simulink model "youbot_no_encoders_joystick_control"  (R2013b)
settings: Solver=ode3  StartTime=0.0  StopTime=inf  FixedStep=0.01  RelTol=1e-3
libraries: vrlib x1, robotica x1
settings Model: Creator=student  LastModifiedBy=student

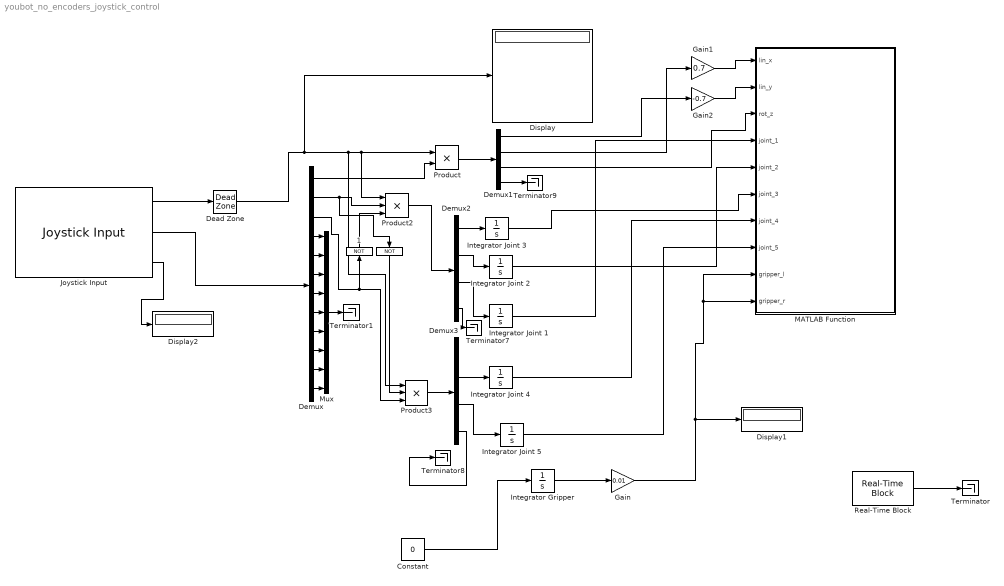
== system youbot_no_encoders_joystick_control ==
  " " : Logic  Operator=NOT  AllPortsSameDT=off  OutDataTypeStr=boolean
  " 1" : Logic  Operator=NOT  AllPortsSameDT=off  OutDataTypeStr=boolean
  Constant : Constant  Value=0
  Dead Zone : DeadZone  LowerValue=-0.1  UpperValue=0.1  SaturateOnIntegerOverflow=on
  Demux : Demux  Outputs=12
  Demux1 : Demux
  Demux2 : Demux
  Demux3 : Demux
  Display : Display
  Display1 : Display
  Display2 : Display
  Gain : Gain  Gain=0.01
  Gain1 : Gain  Gain=0.7
  Gain2 : Gain  Gain=-0.7
  Integrator Gripper : Integrator  LimitOutput=on  UpperSaturationLimit=1  LowerSaturationLimit=0
  "Integrator Joint 5 " : Integrator  InitialCondition=0.12  LimitOutput=on  UpperSaturationLimit=5.64  LowerSaturationLimit=0.12
  "Integrator Joint 1 " : Integrator  InitialCondition=0.02  LimitOutput=on  UpperSaturationLimit=5.84  LowerSaturationLimit=0.02
  Integrator Joint 2 : Integrator  InitialCondition=0.02  LimitOutput=on  UpperSaturationLimit=2.61  LowerSaturationLimit=0.02
  "Integrator Joint 3 " : Integrator  InitialCondition=-0.02  LimitOutput=on  UpperSaturationLimit=-0.02  LowerSaturationLimit=-5.02
  Integrator Joint 4 : Integrator  InitialCondition=0.03  LimitOutput=on  UpperSaturationLimit=3.42  LowerSaturationLimit=0.03
  Joystick Input : vrlib/Joystick Input  joyid=1  adjustports=on  forcefeed=off
  MATLAB Function : MATLAB Function  StartFcn=|  StopFcn=|  TreatAsAtomicUnit=on  mask{youbot_IP=192.168.65.59, youbot_port=11311}
      StartFcn=|
      | %ros_node = rosmatlab.node('KUKA_SIMULINK_CONTROL','192.168.65.59',11311);          
      |  ros_node = rosmatlab.node('KUKA_SIMULINK_CONTROL',youbot_ip, youbot_port);          
      | 
      | % Base                                        
      | 
      |     publisher_na_kuko = rosmatlab.publisher('/cmd_vel','geometry_msgs/Twist',ros_node);                                     
      |     kuka_message = rosmatlab.message('geometry_msgs/Twist',ros_node);                                                       
      |     kuka_message.getLinear.setX(0.0);                                                                                       
      |     kuka_message.getLinear.setY(0);                                                                                         
      |     kuka_message.getLinear.setZ(0);                                                                                         
      |     kuka_message.getAngular.setX(0);                                                                                        
      |     kuka_message.getAngular.setY(0);                                                                                        
      |     kuka_message.getAngular.setZ(0);                                                                                        
      |     publisher_na_kuko.publish(kuka_message);                                                                                
      | 
      | % Arm
      |                                                                                                                             
      | publisher_kuka_arm = rosmatlab.publisher('/arm_1/arm_controller/position_command','brics_actuator/JointPositions',ros_node);
      |                                                                                                                             
      | arm_kuka_message = rosmatlab.message('brics_actuator/JointPositions', ros_node);                                            
      |                                                                                                                             
      | arm_header_message = rosmatlab.message('brics_actuator/Poison', ros_node);                                                  
      |                                                                                                                             
      | joint_1_message =  rosmatlab.message('brics_actuator/JointValue', ros_node);                                                
      |                                                                                                                             
      | joint_2_message= rosmatlab.message('brics_actuator/JointValue', ros_node);                                                  
      |                                                                                                                             
      | joint_3_message = rosmatlab.message('brics_actuator/JointValue', ros_node);                                                 
      |                                                                                                                             
      | joint_4_message = rosmatlab.message('brics_actuator/JointValue', ros_node);                                                 
      |                                                                                                                             
      | joint_5_message = rosmatlab.message('brics_actuator/JointValue', ros_node);                                                 
      |                                                                                                                             
      | arm_header_message.setDescription('Pozdrav iz Simulinka');                                                                  
      | arm_header_message.setOriginator('Simulink');                                                                               
      | arm_header_message.setQos(0.0);                                                                                             
      | arm_kuka_message.setPoisonStamp(arm_header_message);                                                                        
      |                                                                                                                             
      | joint_1_message.setJointUri('arm_joint_1');                                                                                 
      | joint_1_message.setUnit('rad');                                                                                             
      | joint_1_message.setValue(0.02);                                                                                                
      |                                                                                                                             
      | joint_2_message.setJointUri('arm_joint_2');                                                                                 
      | joint_2_message.setUnit('rad');                                                                                             
      | joint_2_message.setValue(0.02);                                                                                                
      |                                                                                                                             
      | joint_3_message.setJointUri('arm_joint_3');                                                                                 
      | joint_3_message.setUnit('rad');                                                                                             
      | joint_3_message.setValue(-0.02);                                                                                                
      |                                                                                                                             
      | joint_4_message.setJointUri('arm_joint_4');                                                                                 
      | joint_4_message.setUnit('rad');                                                                                             
      | joint_4_message.setValue(0.023);                                                                                                
      |                                                                                                                             
      | joint_5_message.setJointUri('arm_joint_5');                                                                                 
      | joint_5_message.setUnit('rad');                                                                                             
      | joint_5_message.setValue(0.12);                                                                                                
      |                                                                                                                             
      | arm_kuka_message.getPositions.add(joint_1_message);                                                                         
      | arm_kuka_message.getPositions.add(joint_2_message);                                                                         
      | arm_kuka_message.getPositions.add(joint_3_message);                                                                         
      | arm_kuka_message.getPositions.add(joint_4_message);                                                                         
      | arm_kuka_message.getPositions.add(joint_5_message);                                                                         
      |                                                                                                                             
      | publisher_kuka_arm.publish(arm_kuka_message);     
      | 
      | % Gripper
      | 
      | gripper_publisher = rosmatlab.publisher('/arm_1/gripper_controller/position_command','brics_actuator/JointPositions',ros_node);
      | 
      | gripper_message = rosmatlab.message('brics_actuator/JointPositions', ros_node);
      | gripper_header_message = rosmatlab.message('brics_actuator/Poison', ros_node);
      | gripper_L_message =  rosmatlab.message('brics_actuator/JointValue', ros_node);
      | gripper_R_message= rosmatlab.message('brics_actuator/JointValue', ros_node);
      | 
      | gripper_header_message.setDescription('Hello Simulink.  Gripper greets you');
      | gripper_header_message.setOriginator('Simulink');
      | gripper_header_message.setQos(0.0);
      | gripper_message.setPoisonStamp(gripper_header_message);
      | 
      | gripper_L_message.setJointUri('gripper_finger_joint_l');
      | gripper_L_message.setUnit('m');
      | gripper_L_message.setValue(0);
      | 
      | gripper_R_message.setJointUri('gripper_finger_joint_r');
      | gripper_R_message.setUnit('m');
      | gripper_R_message.setValue(0);
      | 
      | gripper_message.getPositions.add(gripper_L_message);
      | gripper_message.getPositions.add(gripper_R_message);
      | 
      | gripper_publisher.publish(gripper_message);
      StopFcn=|
      | kuka_message.getLinear.setX(0);         
      | kuka_message.getLinear.setY(0);         
      | kuka_message.getLinear.setZ(0);         
      | kuka_message.getAngular.setX(0);        
      | kuka_message.getAngular.setY(0);        
      | kuka_message.getAngular.setZ(0);        
      | publisher_na_kuko.publish(kuka_message);
      | ros_node.delete                         
      | 
      | clear arm_header_message;
      | clear arm_kuka_message;
      | clear gripper_L_message;
      | clear gripper_R_message;
      | clear gripper_header_message;
      | clear gripper_message;
      | clear gripper_publisher;
      | clear joint_1_message;
      | clear joint_2_message;
      | clear joint_3_message;
      | clear joint_4_message;
      | clear joint_5_message;
      | 
      | clear kuka_message;
      | clear publisher_na_kuko;
      | clear publisher_kuka_arm;
      | 
      | 
      | clear youbot_ip;
      | clear youbot_port;
      | 
      | clear ros_node;
      mask prompts: youbot_IP "Youbot IP address"; youbot_port "Youbot port"
      mask help: Enter the Kuka Youbot IP address and ros core port number.
      mask init:
      | disp('Entered kuka youbot block mask initialization');
      | assignin('base','youbot_ip',youbot_IP);
      | assignin('base','youbot_port',youbot_port);
  Mux : Mux  Inputs=9
  Product : Product
  Product2 : Product  Inputs=3
  Product3 : Product  Inputs=3
  Real-Time Block : robotica/Utilities blocks/Real-Time Block  sync_type=Fixed  sync_time=0.01
  Terminator{,1,7..9} (5 alike) : Terminator
  wires:
  Real-Time Block/1 -> Terminator/1
  Joystick Input/1 -> Dead Zone/1
  Joystick Input/3 -> Display2/1
  Joystick Input/2 -> Demux/1
  Demux/1 -> Product/2
  Demux/2 -> " "/1, Product2/2
  Demux/3 -> Product3/3, " 1"/1
  Demux/4 -> Mux/1
  Demux/5 -> Mux/2
  Demux/6 -> Mux/3
  Demux/7 -> Mux/4
  Demux/8 -> Mux/5
  Demux/9 -> Mux/6
  Demux/10 -> Mux/7
  Demux/11 -> Mux/8
  Demux/12 -> Mux/9
  Mux/1 -> Terminator1/1
  Demux1/3 -> MATLAB Function/3(rot_z)
  Demux1/2 -> Gain1/1
  Demux1/1 -> Gain2/1
  Constant/1 -> Integrator Gripper/1
  Integrator Gripper/1 -> Gain/1
  Gain/1 -> MATLAB Function/9(gripper_l), MATLAB Function/10(gripper_r), Display1/1
  Product/1 -> Demux1/1
  Gain1/1 -> MATLAB Function/1(lin_x)
  Gain2/1 -> MATLAB Function/2(lin_y)
  Dead Zone/1 -> Display/1, Product3/1, Product2/1, Product/1
  Product2/1 -> Demux2/1
  Demux2/3 -> "Integrator Joint 1 "/1
  "Integrator Joint 1 "/1 -> MATLAB Function/4(joint_1)
  Demux2/2 -> Integrator Joint 2/1
  Integrator Joint 2/1 -> MATLAB Function/5(joint_2)
  Demux2/1 -> "Integrator Joint 3 "/1
  "Integrator Joint 3 "/1 -> MATLAB Function/6(joint_3)
  " "/1 -> Product3/2
  " 1"/1 -> Product2/3
  Product3/1 -> Demux3/1
  Demux3/2 -> Integrator Joint 4/1
  Integrator Joint 4/1 -> MATLAB Function/7(joint_4)
  Demux2/4 -> Terminator7/1
  Demux3/3 -> "Integrator Joint 5 "/1
  "Integrator Joint 5 "/1 -> MATLAB Function/8(joint_5)
  Demux3/4 -> Terminator8/1
  Demux1/4 -> Terminator9/1

== matlab function youbot_no_encoders_joystick_control/MATLAB Function ==
  data: lin_x input; lin_y input; rot_z input; joint_1 input; joint_2 input; joint_3 input; joint_4 input; joint_5 input; gripper_l input; gripper_r input
function youbot_control_no_encoders(lin_x,lin_y,rot_z,joint_1,joint_2,joint_3,joint_4,joint_5,gripper_l,gripper_r)

persistent lin_x_old lin_y_old rot_z_old;
persistent joint_1_old joint_2_old joint_3_old joint_4_old joint_5_old ;
persistent gripper_l_old gripper_r_old ; 

if isempty(lin_x_old)  % all initialized at first step
    lin_x_old = 0;
    lin_y_old = 0;
    rot_z_old = 0;
    joint_1_old = 0;
    joint_2_old = 0;
    joint_3_old = 0 ;
    joint_4_old = 0;
    joint_5_old = 0; 
    gripper_l_old = 0;
    gripper_r_old = 0;
    
end

coder.extrinsic('num2str','strcat','evalin');

if lin_x ~= lin_x_old
    ukaz= strcat('kuka_message.getLinear.setX(',num2str(lin_x),')');
    evalin('base', ukaz);
end

if lin_y ~= lin_y_old
    ukaz= strcat('kuka_message.getLinear.setY(',num2str(lin_y),')');
    evalin('base', ukaz);
end

if rot_z ~= rot_z_old
    ukaz= strcat('kuka_message.getAngular.setZ(',num2str(-1.0*rot_z),')');
    evalin('base', ukaz);
end

if (lin_x ~= lin_x_old)||(lin_y ~= lin_y_old)||(rot_z ~= rot_z_old)
    evalin('base','publisher_na_kuko.publish(kuka_message)');
end

if joint_1 ~= joint_1_old
    ukaz= strcat('joint_1_message.setValue(',num2str(joint_1),')');
    evalin('base', ukaz);
end

if joint_2 ~= joint_2_old
    ukaz= strcat('joint_2_message.setValue(',num2str(joint_2),')');
    evalin('base', ukaz);
end

if joint_3 ~= joint_3_old
    ukaz= strcat('joint_3_message.setValue(',num2str(joint_3),')');
    evalin('base', ukaz);
end

if joint_4 ~= joint_4_old
    ukaz= strcat('joint_4_message.setValue(',num2str(joint_4),')');
    evalin('base', ukaz);
end

if joint_5 ~= joint_5_old
    ukaz= strcat('joint_5_message.setValue(',num2str(joint_5),')');
    evalin('base', ukaz);
end

if (joint_1 ~= joint_1_old)||(joint_2 ~= joint_2_old)||(joint_3 ~= joint_3_old)||(joint_4 ~= joint_4_old)||(joint_5 ~= joint_5_old)
    evalin('base','publisher_kuka_arm.publish(arm_kuka_message)');
end

if gripper_l ~= gripper_l_old
    ukaz= strcat('gripper_L_message.setValue(',num2str(gripper_l),')');
    evalin('base', ukaz);
end

if gripper_r ~= gripper_r_old
    ukaz= strcat('gripper_R_message.setValue(',num2str(gripper_r),')');
    evalin('base', ukaz);
end

if (gripper_l ~= gripper_l_old)||(gripper_r ~= gripper_r_old)
    evalin('base','gripper_publisher.publish(gripper_message)');
end


lin_x_old = lin_x;
lin_y_old = lin_y;
rot_z_old = rot_z;
joint_1_old = joint_1;
joint_2_old = joint_2;
joint_3_old = joint_3;
joint_4_old = joint_4;
joint_5_old = joint_5;
gripper_l_old = gripper_l;
gripper_r_old = gripper_r;

% joint_positions = zeros(7,1);
% joint_speeds = zeros(7,1);
% joint_positions = evalin('base','arm_position');
% joint_speeds = evalin('base','arm_velocities');
% 
% base_positions = zeros(8,1);
% base_speeds = zeros(8,1);
% base_positions = evalin('base','base_position');
% base_speeds = evalin('base','base_velocities');
% 
% joint_1_out = [joint_positions(1); joint_speeds(1)];
% joint_2_out = [joint_positions(2); joint_speeds(2)];
% joint_3_out = [joint_positions(3); joint_speeds(3)];
% joint_4_out = [joint_positions(4); joint_speeds(4)];
% joint_5_out = [joint_positions(5); joint_speeds(5)];
% gripper_L_out = [joint_positions(6); joint_speeds(6)];
% gripper_R_out = [joint_positions(7); joint_speeds(7)];
% 
% wheel_FL_out = [base_positions(1); base_speeds(1)];
% wheel_FR_out = [base_positions(2); base_speeds(2)];
% wheel_BL_out = [base_positions(3); base_speeds(3)];
% wheel_BR_out = [base_positions(4); base_speeds(4)];
